simulink model "xdd_zy2_2"  (R2023b)
settings: Solver=VariableStepAuto  StartTime=0.0  StopTime=30  RelTol=1e-3
libraries: commrandsrc3 x1
settings Model: Creator=Bricksburg-Akataka  LastModifiedBy=Bricksburg-Akataka

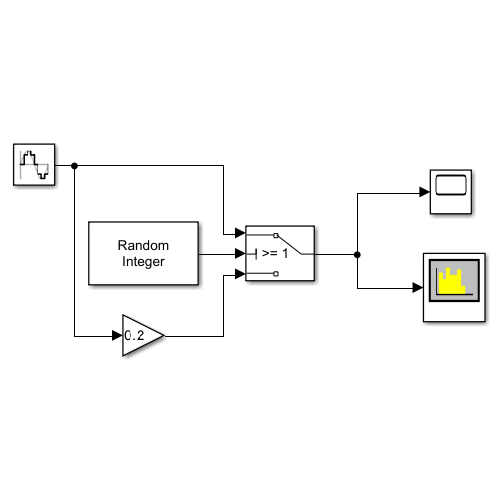
[thumbnail: Simulink's stored preview of the top-level diagram]
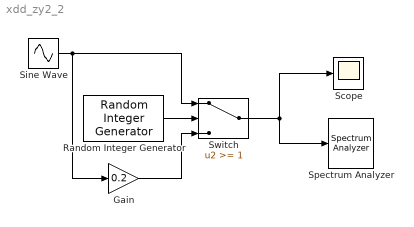
== system xdd_zy2_2 ==
  Gain : Gain  Gain=0.2
  Random Integer Generator : commrandsrc3/Random Integer Generator  SetSize=2  SeedSource=Auto  Seed=0  SampleTime=1  SamplesPerFrame=1  OutputDataType=double  SimulateUsing=Interpreted execution
  Scope : Scope
  Sine Wave : Sin  Frequency=2*pi*10  SampleTime=1/100
  Spectrum Analyzer : SpectrumAnalyzer  WindowPosition=[777.000000,120.000000,800.000000,500.000000,]  ScopeFrameLocation=window  YLimits=[-158.43800339,-69.4633435]
  Switch : Switch  Threshold=1  SaturateOnIntegerOverflow=off  InputSameDT=off
  wires:
  Random Integer Generator/1 -> Switch/2
  Gain/1 -> Switch/3
  Sine Wave/1 -> Gain/1, Switch/1
  Switch/1 -> Scope/1, Spectrum Analyzer/1
